simulink model "PWM"  (R2017a)
settings: Solver=VariableStepAuto  StartTime=0.0  StopTime=0.12  RelTol=1e-3
libraries: simulink x2, powerlib_meascontrol x1
settings Model: Creator=Michy  LastModifiedBy=Michy

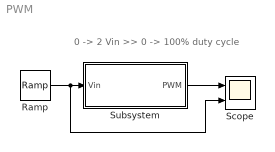
== system PWM ==
  note: 0 -> 2 Vin >> 0 -> 100% duty cycle
  Ramp : simulink/Sources/Ramp  slope=50  start=0  X0=-3
  Scope : Scope  NumInputPorts=2
  Subsystem : Subsystem
  wires:
  Ramp/1 -> Scope/2, Subsystem/1(Vin)
  Subsystem/1(PWM) -> Scope/1

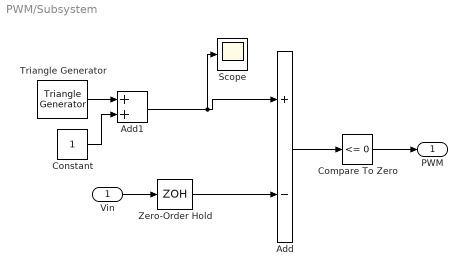
== system PWM/Subsystem ==
  Vin : Inport
  Add : Sum  Inputs=+-
  Add1 : Sum
  Compare To Zero : simulink/Logic and Bit Operations/Compare To Zero  relop=<=  OutDataTypeStr=boolean
  Constant : Constant
  Scope : Scope
  Triangle Generator : powerlib_meascontrol/Pulse & Signal Generators/Triangle Generator  Freq=1e3  Phase=90  Ts=0
  Zero-Order Hold : ZeroOrderHold  SampleTime=-1
  PWM : Outport
  wires:
  Vin/1 -> Zero-Order Hold/1
  Zero-Order Hold/1 -> Add/2
  Add/1 -> Compare To Zero/1
  Compare To Zero/1 -> PWM/1
  Triangle Generator/1 -> Add1/1
  Add1/1 -> Scope/1, Add/1
  Constant/1 -> Add1/2
